simulink model "exp8_4"  (R2023a)
settings: Solver=VariableStepAuto  StartTime=0.0  StopTime=50  RelTol=1e-3
settings Model: Creator=Lenovo  LastModifiedBy=zt

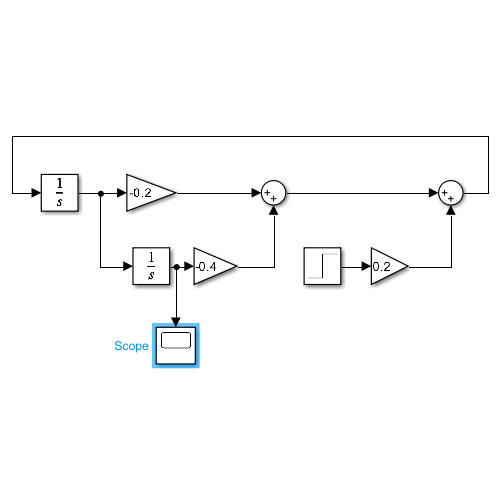
[thumbnail: Simulink's stored preview of the top-level diagram]
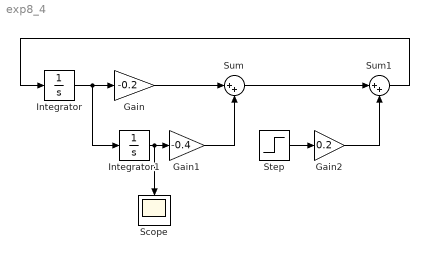
== system exp8_4 ==
  Gain : Gain  Gain=-0.2
  Gain1 : Gain  Gain=-0.4
  Gain2 : Gain  Gain=0.2
  Integrator : Integrator
  Integrator1 : Integrator
  Scope : Scope
  Step : Step  SampleTime=0
  Sum : Sum  Inputs=|++
  Sum1 : Sum  Inputs=|++
  wires:
  Integrator/1 -> Integrator1/1, Gain/1
  Integrator1/1 -> Scope/1, Gain1/1
  Gain/1 -> Sum/1
  Gain1/1 -> Sum/2
  Step/1 -> Gain2/1
  Sum/1 -> Sum1/1
  Gain2/1 -> Sum1/2
  Sum1/1 -> Integrator/1
